simulink model "Test_SimFEAdapter"  (Simulink 7.4)
settings: Solver=FixedStepDiscrete  StartTime=0.0  StopTime=inf  FixedStep=samplePeriod  RelTol=1e-3  AbsTol=1e-6
PreLoadFcn:
  | initializeSimulation
InitFcn:
  | clear('all');
  | initializeSimulation;
values from neighbouring files (symbols this model uses):
  damperA = 0    [initializeSimulation.m]
  damperB = 0    [initializeSimulation.m]
  damperC = 0    [initializeSimulation.m]
  damperCanon = 1    [initializeSimulation.m]
  flowCanon = 3.85    [initializeSimulation.m]
  forceCanon = 1    [initializeSimulation.m]
  frictionA = 0    [initializeSimulation.m]
  frictionB = 0    [initializeSimulation.m]
  frictionC = 0    [initializeSimulation.m]
  gasConstant = 1.8    [initializeSimulation.m]
  lengthCanon = 1    [initializeSimulation.m]
  massA = 4.2    [initializeSimulation.m]
  massB = 2.5    [initializeSimulation.m]
  massC = 2.5    [initializeSimulation.m]
  massCanon = 0.002588    [initializeSimulation.m]
  maxDisplA = (stroke2A + endLength2A) * lengthCanon    (= 22)    [initializeSimulation.m]
  maxDisplB = (stroke2B + endLength2B) * lengthCanon    (= 42)    [initializeSimulation.m]
  maxDisplC = (stroke2C + endLength2C) * lengthCanon    (= 72)    [initializeSimulation.m]
  maxOilVolume = volume * (1 - (precharge/supplyPress)^(1/gasConstant))    (= 10.5071802963)    [initializeSimulation.m]
  maxVelocA = (maxFlowA * flowCanon / (area1A * areaCanon)) / velocCanon    [initializeSimulation.m]
  maxVelocB = (maxFlowB * flowCanon / (area1B * areaCanon)) / velocCanon    [initializeSimulation.m]
  maxVelocC = (maxFlowC * flowCanon / (area1C * areaCanon)) / velocCanon    [initializeSimulation.m]
  minDisplA = -(stroke1A + endLength1A) * lengthCanon    (= -22)    [initializeSimulation.m]
  minDisplB = -(stroke1B + endLength1B) * lengthCanon    (= -42)    [initializeSimulation.m]
  minDisplC = -(stroke1C + endLength1C) * lengthCanon    (= -72)    [initializeSimulation.m]
  minVelocA = -(maxFlowA * flowCanon / (area2A * areaCanon)) / velocCanon    [initializeSimulation.m]
  minVelocB = -(maxFlowB * flowCanon / (area2B * areaCanon)) / velocCanon    [initializeSimulation.m]
  minVelocC = -(maxFlowC * flowCanon / (area2C * areaCanon)) / velocCanon    [initializeSimulation.m]
  nAct = 8    [initializeSimulation.m]
  nAdcU = 12    [initializeSimulation.m]
  nDinp = 4    [initializeSimulation.m]
  nDout = 4    [initializeSimulation.m]
  nDucU = 8    [initializeSimulation.m]
  nEncU = 2    [initializeSimulation.m]
  precharge = 1000    [initializeSimulation.m]
  pumpFlow = 1e10    (= 10000000000)    [initializeSimulation.m]
  returnPress = 50    [initializeSimulation.m]
  staticForceA = 0    [initializeSimulation.m]
  staticForceB = 0    [initializeSimulation.m]
  staticForceC = 0    [initializeSimulation.m]
  supplyPress = 3000    [initializeSimulation.m]
  velocCanon = 1    [initializeSimulation.m]
  volume = accumVolume * accumNumber    (= 23)    [initializeSimulation.m]
  volumeCanon = 231    [initializeSimulation.m]
  yieldDisplA = 0.1    [initializeSimulation.m]
  yieldDisplB = 0.1    [initializeSimulation.m]
  yieldDisplC = 0.1    [initializeSimulation.m]
undefined symbols (not defined in the file or in its folder): DiscIntNeverNeededParam
(part 1 of 3)
settings Model: Creator=Andreas Schellenberg  LastModifiedBy=Andreas  ExtModeTrigMode=oneshot  ExtModeArmWhenConnect=off  ExtModeAutoUpdateStatusClock=off
settings DataIOCC: SaveOutput=off  SaveTime=off  SignalLoggingName=sigsOut
settings OptimizationCC: EnforceIntegerDowncast=off  InitFltsAndDblsToZero=on
settings DebuggingCC: SaveWithParameterizedLinksMsg=none  CheckSSInitialOutputMsg=off  SolverPrmCheckMsg=none  MultiTaskDSMMsg=warning  MultiTaskCondExecSysMsg=none  StrictBusMsg=None
settings HardwareCC: TargetUnknown=on
settings SFSimCC: SimCustomHeaderCode="#include \"PredictorCorrector.h\""  SimUserSources=PredictorCorrector.c
settings RTWCC: IncludeERTFirstTime=on
settings GRTTargetCC: TargetFcnLib=ansi_tfl_tmw.mat

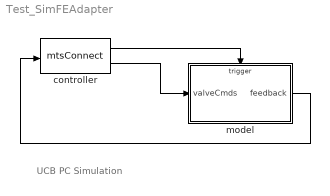
== system Test_SimFEAdapter ==
  note: UCB PC Simulation
  controller : S-Function  FunctionName=mtsConnect  Parameters='127.0.0.1',5002,nUDPInp,nUDPOut  EnableBusSupport=off
  model : Subsystem  TreatAsAtomicUnit=on
  wires:
  model/1(feedback) -> controller/1
  controller/2 -> model/1(valveCmds)
  controller/1 -> model/Trigger

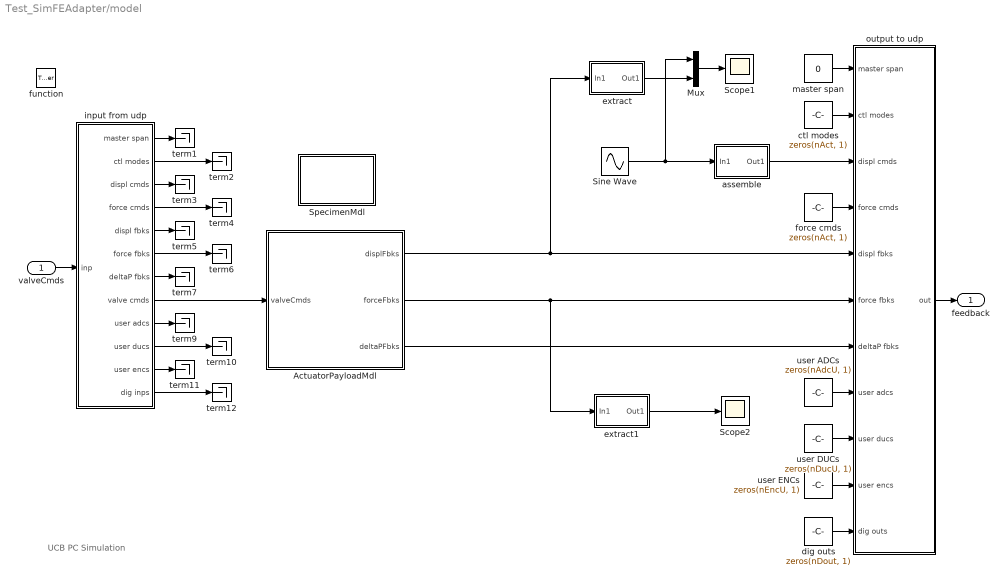
== system Test_SimFEAdapter/model ==
  note: UCB PC Simulation
  valveCmds : Inport  OutDataType=sfix(16)  OutScaling=2^0
  function : TriggerPort  TriggerType=function-call
  ActuatorPayloadMdl : Subsystem
  Mux : Mux  Inputs=2
  Scope1 : Scope
      settings: TimeRange=15  YMin=-1.5  YMax=1.5
  Scope2 : Scope
      settings: TimeRange=15  YMin=-6  YMax=8
  Sine Wave : Sin  Amplitude=1  Bias=0  Frequency=pi  Phase=0  Samples=10  Offset=0
  SpecimenMdl : Subsystem
      mask Display: fprintf('Test\nSpecimen');
  assemble : Subsystem  mask(to Actuators){id=1, size=nAct}
      mask prompts: id "Index Vector: id"; size "Vector Size: size"
      mask help: To select to which actuator(s) the signals are going to
      mask Display: disp('Assemble')
  ctl modes : Constant  Value=zeros(nAct, 1)  OutDataType=sfix(16)  OutScaling=2^0
  dig outs : Constant  Value=zeros(nDout, 1)  OutDataTypeMode=uint32  OutDataType=sfix(16)  OutScaling=2^0  OutDataTypeStr=uint32
  extract : Subsystem  mask(from Actuators){id=1, size=nAct}
      mask prompts: id "Index Vector: id"; size "Vector Size: size"
      mask help: To select from which actuator(s) the signals are coming from
      mask Display: disp('Extract')
  extract1 : Subsystem  mask(from Actuators){id=1, size=nAct}
      mask prompts: id "Index Vector: id"; size "Vector Size: size"
      mask help: To select from which actuator(s) the signals are coming from
      mask Display: disp('Extract')
  force cmds : Constant  Value=zeros(nAct, 1)  OutDataType=sfix(16)  OutScaling=2^0
  input from udp : Subsystem
  master span : Constant  Value=0  OutDataType=sfix(16)  OutScaling=2^0
  output to udp : Subsystem
  term{1..7,9..12} (11 alike) : Terminator
  user ADCs : Constant  Value=zeros(nAdcU, 1)  OutDataType=sfix(16)  OutScaling=2^0
  user DUCs : Constant  Value=zeros(nDucU, 1)  OutDataType=sfix(16)  OutScaling=2^0
  user ENCs : Constant  Value=zeros(nEncU, 1)  OutDataType=sfix(16)  OutScaling=2^0
  feedback : Outport  OutDataType=sfix(16)  OutScaling=2^0
  wires:
  input from udp/3(displ cmds) -> term3/1
  input from udp/1(master span) -> term1/1
  input from udp/6(force fbks) -> term6/1
  input from udp/10(user ducs) -> term10/1
  input from udp/12(dig inps) -> term12/1
  input from udp/2(ctl modes) -> term2/1
  input from udp/4(force cmds) -> term4/1
  input from udp/5(displ fbks) -> term5/1
  input from udp/7(deltaP fbks) -> term7/1
  input from udp/9(user adcs) -> term9/1
  input from udp/11(user encs) -> term11/1
  valveCmds/1 -> input from udp/1(inp)
  master span/1 -> output to udp/1(master span)
  ctl modes/1 -> output to udp/2(ctl modes)
  assemble/1(Out1) -> output to udp/3(displ cmds)
  force cmds/1 -> output to udp/4(force cmds)
  user ADCs/1 -> output to udp/8(user adcs)
  user DUCs/1 -> output to udp/9(user ducs)
  user ENCs/1 -> output to udp/10(user encs)
  dig outs/1 -> output to udp/11(dig outs)
  output to udp/1(out) -> feedback/1
  ActuatorPayloadMdl/1(displFbks) -> output to udp/5(displ fbks), extract/1(In1)
  ActuatorPayloadMdl/2(forceFbks) -> output to udp/6(force fbks), extract1/1(In1)
  ActuatorPayloadMdl/3(deltaPFbks) -> output to udp/7(deltaP fbks)
  input from udp/8(valve cmds) -> ActuatorPayloadMdl/1(valveCmds)
  Sine Wave/1 -> assemble/1(In1), Mux/1
  Mux/1 -> Scope1/1
  extract/1(Out1) -> Mux/2
  extract1/1(Out1) -> Scope2/1

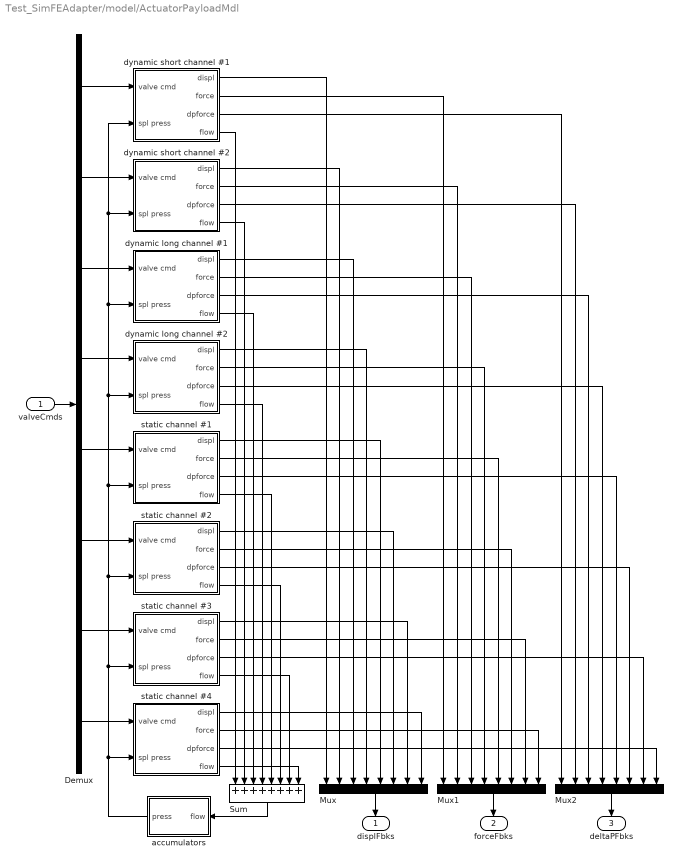
== system Test_SimFEAdapter/model/ActuatorPayloadMdl ==
  valveCmds : Inport  OutDataType=sfix(16)  OutScaling=2^0
  Demux : Demux  Outputs=nAct
  Mux : Mux  Inputs=nAct
  Mux1 : Mux  Inputs=nAct
  Mux2 : Mux  Inputs=nAct
  Sum : Sum  Inputs=++++++++  OutDataType=sfix(16)  OutScaling=2^0  SaturateOnIntegerOverflow=on
  accumulators : Subsystem
  dynamic long channel #1 : Subsystem
  dynamic long channel #2 : Subsystem
  dynamic short channel #1 : Subsystem
  dynamic short channel #2 : Subsystem
  static channel #1 : Subsystem
  static channel #2 : Subsystem
  static channel #3 : Subsystem
  static channel #4 : Subsystem
  displFbks : Outport  OutDataType=sfix(16)  OutScaling=2^0
  forceFbks : Outport  Port=2  OutDataType=sfix(16)  OutScaling=2^0
  deltaPFbks : Outport  Port=3  OutDataType=sfix(16)  OutScaling=2^0
  wires:
  Demux/1 -> dynamic short channel #1/1(valve cmd)
  Demux/3 -> dynamic long channel #1/1(valve cmd)
  Demux/2 -> dynamic short channel #2/1(valve cmd)
  dynamic short channel #1/4(flow) -> Sum/1
  dynamic short channel #2/4(flow) -> Sum/2
  dynamic long channel #1/4(flow) -> Sum/3
  Sum/1 -> accumulators/1(flow)
  Demux/4 -> dynamic long channel #2/1(valve cmd)
  Demux/5 -> static channel #1/1(valve cmd)
  Demux/6 -> static channel #2/1(valve cmd)
  Demux/7 -> static channel #3/1(valve cmd)
  Demux/8 -> static channel #4/1(valve cmd)
  dynamic long channel #2/4(flow) -> Sum/4
  static channel #1/4(flow) -> Sum/5
  static channel #2/4(flow) -> Sum/6
  static channel #3/4(flow) -> Sum/7
  static channel #4/4(flow) -> Sum/8
  accumulators/1(press) -> static channel #4/2(spl press), static channel #3/2(spl press), static channel #2/2(spl press), static channel #1/2(spl press), dynamic long channel #2/2(spl press), dynamic long channel #1/2(spl press), dynamic short channel #2/2(spl press), dynamic short channel #1/2(spl press)
  dynamic short channel #1/1(displ) -> Mux/1
  dynamic short channel #2/1(displ) -> Mux/2
  dynamic long channel #1/1(displ) -> Mux/3
  dynamic long channel #2/1(displ) -> Mux/4
  static channel #1/1(displ) -> Mux/5
  static channel #2/1(displ) -> Mux/6
  static channel #3/1(displ) -> Mux/7
  static channel #4/1(displ) -> Mux/8
  dynamic short channel #1/2(force) -> Mux1/1
  dynamic short channel #2/2(force) -> Mux1/2
  dynamic long channel #1/2(force) -> Mux1/3
  dynamic long channel #2/2(force) -> Mux1/4
  static channel #1/2(force) -> Mux1/5
  static channel #2/2(force) -> Mux1/6
  static channel #3/2(force) -> Mux1/7
  static channel #4/2(force) -> Mux1/8
  dynamic short channel #1/3(dpforce) -> Mux2/1
  dynamic short channel #2/3(dpforce) -> Mux2/2
  dynamic long channel #1/3(dpforce) -> Mux2/3
  dynamic long channel #2/3(dpforce) -> Mux2/4
  static channel #1/3(dpforce) -> Mux2/5
  static channel #2/3(dpforce) -> Mux2/6
  static channel #3/3(dpforce) -> Mux2/7
  static channel #4/3(dpforce) -> Mux2/8
  valveCmds/1 -> Demux/1
  Mux/1 -> displFbks/1
  Mux1/1 -> forceFbks/1
  Mux2/1 -> deltaPFbks/1

== system Test_SimFEAdapter/model/SpecimenMdl ==
  Scope3 : Scope
      settings: TimeRange=14  YMin=-2  YMax=2  SaveName=ScopeData2
  Specimen #1 : S-Function  FunctionName=SFun_SimFEAdapter  Parameters=ipAddr,ipPort,dataSize  EnableBusSupport=off  mask(GenericClient Element){ipAddr=127.0.0.1, ipPort=44000, dataSize=256}
      mask prompts: ipAddr "IP Address of Adapter Element"; ipPort "IP Port Number of Adapter Element"; dataSize "Size of Data Arrays"
      mask Display: disp('SimFE\nAdapter');
  Terminator : Terminator
  assemble1 : Subsystem  mask(to Actuators){id=1, size=nAct}
      mask prompts: id "Index Vector: id"; size "Vector Size: size"
      mask help: To select to which actuator(s) the signals are going to
      mask Display: disp('Assemble')
  assemble2 : Subsystem  mask(to Actuators){id=1, size=nAct}
      mask prompts: id "Index Vector: id"; size "Vector Size: size"
      mask help: To select to which actuator(s) the signals are going to
      mask Display: disp('Assemble')
  extract2 : Subsystem  mask(from Actuators){id=1, size=nAct}
      mask prompts: id "Index Vector: id"; size "Vector Size: size"
      mask help: To select from which actuator(s) the signals are coming from
      mask Display: disp('Extract')
  from Actuators : Subsystem
  to LoadCells : Subsystem
  wires:
  from Actuators/1(ctrlDisp) -> extract2/1(In1)
  extract2/1(Out1) -> Specimen #1/1
  Specimen #1/1 -> assemble2/1(In1)
  Specimen #1/2 -> assemble1/1(In1), Scope3/1
  assemble2/1(Out1) -> Terminator/1
  assemble1/1(Out1) -> to LoadCells/1(daqForce)

== system Test_SimFEAdapter/model/assemble ==
  In1 : Inport  OutDataType=sfix(16)  OutScaling=2^0
  Assignment : Assignment  OutputInitialize=Specify size for each dimension in table  IndexOptions=Index vector (port)  Indices=1  OutputSizes=nAct
  Constant : Constant  Value=id  OutDataType=sfix(16)  OutScaling=2^0
  Out1 : Outport  OutDataType=sfix(16)  OutScaling=2^0
  wires:
  Constant/1 -> Assignment/2
  Assignment/1 -> Out1/1
  In1/1 -> Assignment/1

== system Test_SimFEAdapter/model/extract ==
  In1 : Inport  OutDataType=sfix(16)  OutScaling=2^0
  Selector : Selector  InputPortWidth=size  IndexOptions=Index vector (dialog)  Indices=id  OutputSizes=1
  Out1 : Outport  OutDataType=sfix(16)  OutScaling=2^0
  wires:
  Selector/1 -> Out1/1
  In1/1 -> Selector/1

== system Test_SimFEAdapter/model/extract1 ==
  In1 : Inport  OutDataType=sfix(16)  OutScaling=2^0
  Selector : Selector  InputPortWidth=size  IndexOptions=Index vector (dialog)  Indices=id  OutputSizes=1
  Out1 : Outport  OutDataType=sfix(16)  OutScaling=2^0
  wires:
  Selector/1 -> Out1/1
  In1/1 -> Selector/1

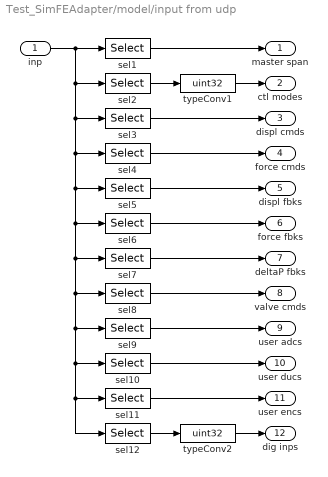
== system Test_SimFEAdapter/model/input from udp ==
  inp : Inport  OutDataType=sfix(16)  OutScaling=2^0
  sel1 : Selector  InputPortWidth=nUDPOut  IndexOptions=Index vector (dialog)  Indices=[0]+1  OutputSizes=1
  sel10 : Selector  InputPortWidth=nUDPOut  IndexOptions=Index vector (dialog)  Indices=[1:nDucU]+1+7*nAct+nAdcU  OutputSizes=1
  sel11 : Selector  InputPortWidth=nUDPOut  IndexOptions=Index vector (dialog)  Indices=[1:nEncU]+1+7*nAct+nAdcU+nDucU  OutputSizes=1
  sel12 : Selector  InputPortWidth=nUDPOut  IndexOptions=Index vector (dialog)  Indices=[1:nDinp]+1+7*nAct+nAdcU+nDucU+nEncU  OutputSizes=1
  sel2 : Selector  InputPortWidth=nUDPOut  IndexOptions=Index vector (dialog)  Indices=[1:nAct]+1+0*nAct  OutputSizes=1
  sel3 : Selector  InputPortWidth=nUDPOut  IndexOptions=Index vector (dialog)  Indices=[1:nAct]+1+1*nAct  OutputSizes=1
  sel4 : Selector  InputPortWidth=nUDPOut  IndexOptions=Index vector (dialog)  Indices=[1:nAct]+1+2*nAct  OutputSizes=1
  sel5 : Selector  InputPortWidth=nUDPOut  IndexOptions=Index vector (dialog)  Indices=[1:nAct]+1+3*nAct  OutputSizes=1
  sel6 : Selector  InputPortWidth=nUDPOut  IndexOptions=Index vector (dialog)  Indices=[1:nAct]+1+4*nAct  OutputSizes=1
  sel7 : Selector  InputPortWidth=nUDPOut  IndexOptions=Index vector (dialog)  Indices=[1:nAct]+1+5*nAct  OutputSizes=1
  sel8 : Selector  InputPortWidth=nUDPOut  IndexOptions=Index vector (dialog)  Indices=[1:nAct]+1+6*nAct  OutputSizes=1
  sel9 : Selector  InputPortWidth=nUDPOut  IndexOptions=Index vector (dialog)  Indices=[1:nAdcU]+1+7*nAct  OutputSizes=1
  typeConv1 : DataTypeConversion  OutDataTypeMode=uint32  OutDataType=sfix(16)  OutScaling=2^0  OutDataTypeStr=uint32  SaturateOnIntegerOverflow=on  RndMeth=Zero
  typeConv2 : DataTypeConversion  OutDataTypeMode=uint32  OutDataType=sfix(16)  OutScaling=2^0  OutDataTypeStr=uint32  SaturateOnIntegerOverflow=on  RndMeth=Zero
  master span : Outport  OutDataType=sfix(16)  OutScaling=2^0
  ctl modes : Outport  Port=2  OutDataType=sfix(16)  OutScaling=2^0
  displ cmds : Outport  Port=3  OutDataType=sfix(16)  OutScaling=2^0
  force cmds : Outport  Port=4  OutDataType=sfix(16)  OutScaling=2^0
  displ fbks : Outport  Port=5  OutDataType=sfix(16)  OutScaling=2^0
  force fbks : Outport  Port=6  OutDataType=sfix(16)  OutScaling=2^0
  deltaP fbks : Outport  Port=7  OutDataType=sfix(16)  OutScaling=2^0
  valve cmds : Outport  Port=8  OutDataType=sfix(16)  OutScaling=2^0
  user adcs : Outport  Port=9  OutDataType=sfix(16)  OutScaling=2^0
  user ducs : Outport  Port=10  OutDataType=sfix(16)  OutScaling=2^0
  user encs : Outport  Port=11  OutDataType=sfix(16)  OutScaling=2^0
  dig inps : Outport  Port=12  OutDataType=sfix(16)  OutScaling=2^0
  wires:
  sel1/1 -> master span/1
  sel2/1 -> typeConv1/1
  sel3/1 -> displ cmds/1
  sel4/1 -> force cmds/1
  sel5/1 -> displ fbks/1
  sel6/1 -> force fbks/1
  sel7/1 -> deltaP fbks/1
  sel8/1 -> valve cmds/1
  sel9/1 -> user adcs/1
  sel10/1 -> user ducs/1
  sel11/1 -> user encs/1
  sel12/1 -> typeConv2/1
  inp/1 -> sel1/1, sel2/1, sel3/1, sel11/1, sel12/1, sel10/1, sel9/1, sel8/1, sel7/1, sel6/1, sel5/1, sel4/1
  typeConv1/1 -> ctl modes/1
  typeConv2/1 -> dig inps/1

== system Test_SimFEAdapter/model/output to udp ==
  master span : Inport  OutDataType=sfix(16)  OutScaling=2^0
  ctl modes : Inport  Port=2  OutDataType=sfix(16)  OutScaling=2^0
  displ cmds : Inport  Port=3  OutDataType=sfix(16)  OutScaling=2^0
  force cmds : Inport  Port=4  OutDataType=sfix(16)  OutScaling=2^0
  displ fbks : Inport  Port=5  OutDataType=sfix(16)  OutScaling=2^0
  force fbks : Inport  Port=6  OutDataType=sfix(16)  OutScaling=2^0
  deltaP fbks : Inport  Port=7  OutDataType=sfix(16)  OutScaling=2^0
  user adcs : Inport  Port=8  OutDataType=sfix(16)  OutScaling=2^0
  user ducs : Inport  Port=9  OutDataType=sfix(16)  OutScaling=2^0
  user encs : Inport  Port=10  OutDataType=sfix(16)  OutScaling=2^0
  dig outs : Inport  Port=11  OutDataType=sfix(16)  OutScaling=2^0
  Mux : Mux  Inputs=11
  typeConv1 : DataTypeConversion  OutDataTypeMode=double  OutDataType=sfix(16)  OutScaling=2^0  OutDataTypeStr=double  SaturateOnIntegerOverflow=on  RndMeth=Zero
  typeConv2 : DataTypeConversion  OutDataTypeMode=double  OutDataType=sfix(16)  OutScaling=2^0  OutDataTypeStr=double  SaturateOnIntegerOverflow=on  RndMeth=Zero
  out : Outport  OutDataType=sfix(16)  OutScaling=2^0
  wires:
  typeConv2/1 -> Mux/11
  dig outs/1 -> typeConv2/1
  user encs/1 -> Mux/10
  user ducs/1 -> Mux/9
  user adcs/1 -> Mux/8
  deltaP fbks/1 -> Mux/7
  force fbks/1 -> Mux/6
  displ fbks/1 -> Mux/5
  force cmds/1 -> Mux/4
  master span/1 -> Mux/1
  displ cmds/1 -> Mux/3
  ctl modes/1 -> typeConv1/1
  Mux/1 -> out/1
  typeConv1/1 -> Mux/2

== system Test_SimFEAdapter/model/ActuatorPayloadMdl/accumulators ==
  flow : Inport  OutDataType=sfix(16)  OutScaling=2^0
  Sum : Sum  Inputs=+-|  OutDataType=sfix(16)  OutScaling=2^0  SaturateOnIntegerOverflow=on  InputSameDT=on  OutDataTypeStr=Inherit: Same as first input
  Sum1 : Sum  Inputs=+-|  OutDataType=sfix(16)  OutScaling=2^0  SaturateOnIntegerOverflow=on  InputSameDT=on  OutDataTypeStr=Inherit: Same as first input
  bottle volume : Constant  Value=volume*volumeCanon  OutDataType=sfix(16)  OutScaling=2^0
  flowCanon : Gain  Gain=flowCanon  ParameterDataType=sfix(16)  ParameterScaling=2^0  OutDataType=sfix(16)  OutScaling=2^0  SaturateOnIntegerOverflow=on  OutDataTypeStr=Inherit: Same as input  ParamDataTypeStr=Inherit: Same as input
  gas constant : Constant  Value=gasConstant  OutDataType=sfix(16)  OutScaling=2^0
  initial condition : UnitDelay  X0=supplyPress  SampleTime=-1
  integrator : DiscreteIntegrator  InitialCondition=maxOilVolume*volumeCanon  SampleTime=-1  OutDataType=sfix(16)  OutScaling=2^0  LimitOutput=on  UpperSaturationLimit=maxOilVolume*volumeCanon  LowerSaturationLimit=0  ICPrevOutput=DiscIntNeverNeededParam  ICPrevScaledInput=DiscIntNeverNeededParam
  power : Math  Operator=pow  OutDataType=sfix(16)  OutScaling=2^0  SaturateOnIntegerOverflow=on
  precharge : Gain  Gain=precharge  ParameterDataType=sfix(16)  ParameterScaling=2^0  OutDataType=sfix(16)  OutScaling=2^0  SaturateOnIntegerOverflow=on  OutDataTypeStr=Inherit: Same as input  ParamDataTypeStr=Inherit: Same as input
  pump flow : Constant  Value=pumpFlow  OutDataType=sfix(16)  OutScaling=2^0
  quotient : Product  Inputs=*/  OutDataType=sfix(16)  OutScaling=2^0  SaturateOnIntegerOverflow=on  InputSameDT=on  OutDataTypeStr=Inherit: Same as first input
  press : Outport  OutDataType=sfix(16)  OutScaling=2^0
  wires:
  initial condition/1 -> press/1
  flowCanon/1 -> integrator/1
  flow/1 -> Sum/2
  integrator/1 -> Sum1/2  "current oil volume"
  quotient/1 -> power/1
  Sum1/1 -> quotient/2  "current gas volume"
  precharge/1 -> initial condition/1
  power/1 -> precharge/1
  gas constant/1 -> power/2
  bottle volume/1 -> quotient/1, Sum1/1
  Sum/1 -> flowCanon/1
  pump flow/1 -> Sum/1

== system Test_SimFEAdapter/model/ActuatorPayloadMdl/dynamic long channel #1 ==
  valve cmd : Inport  OutDataType=sfix(16)  OutScaling=2^0
  spl press : Inport  Port=2  OutDataType=sfix(16)  OutScaling=2^0
  actuator/valve  model : Subsystem
      mask Type: Inverse Actuator
  payload : Subsystem
  return pressure : Constant  Value=returnPress  OutDataType=sfix(16)  OutScaling=2^0
  displ : Outport  OutDataType=sfix(16)  OutScaling=2^0
  force : Outport  Port=2  OutDataType=sfix(16)  OutScaling=2^0
  dpforce : Outport  Port=3  OutDataType=sfix(16)  OutScaling=2^0
  flow : Outport  Port=4  OutDataType=sfix(16)  OutScaling=2^0
  wires:
  payload/2(veloc) -> actuator/valve  model/3(veloc)
  payload/1(displ) -> displ/1, actuator/valve  model/2(displ)
  valve cmd/1 -> actuator/valve  model/1(cmd)
  return pressure/1 -> actuator/valve  model/5(rtn press)
  spl press/1 -> actuator/valve  model/4(spl press)
  actuator/valve  model/2(flow) -> flow/1
  actuator/valve  model/1(force) -> force/1, dpforce/1, payload/1(force)

== system Test_SimFEAdapter/model/ActuatorPayloadMdl/dynamic long channel #2 ==
  valve cmd : Inport  OutDataType=sfix(16)  OutScaling=2^0
  spl press : Inport  Port=2  OutDataType=sfix(16)  OutScaling=2^0
  actuator/valve  model : Subsystem
      mask Type: Inverse Actuator
  payload : Subsystem
  return pressure : Constant  Value=returnPress  OutDataType=sfix(16)  OutScaling=2^0
  displ : Outport  OutDataType=sfix(16)  OutScaling=2^0
  force : Outport  Port=2  OutDataType=sfix(16)  OutScaling=2^0
  dpforce : Outport  Port=3  OutDataType=sfix(16)  OutScaling=2^0
  flow : Outport  Port=4  OutDataType=sfix(16)  OutScaling=2^0
  wires:
  actuator/valve  model/1(force) -> dpforce/1, force/1, payload/1(force)
  actuator/valve  model/2(flow) -> flow/1
  spl press/1 -> actuator/valve  model/4(spl press)
  return pressure/1 -> actuator/valve  model/5(rtn press)
  valve cmd/1 -> actuator/valve  model/1(cmd)
  payload/1(displ) -> actuator/valve  model/2(displ), displ/1
  payload/2(veloc) -> actuator/valve  model/3(veloc)

== system Test_SimFEAdapter/model/ActuatorPayloadMdl/dynamic short channel #1 ==
  valve cmd : Inport  OutDataType=sfix(16)  OutScaling=2^0
  spl press : Inport  Port=2  OutDataType=sfix(16)  OutScaling=2^0
  actuator/valve  model : Subsystem
      mask Type: Inverse Actuator
  payload : Subsystem
  return pressure : Constant  Value=returnPress  OutDataType=sfix(16)  OutScaling=2^0
  displ : Outport  OutDataType=sfix(16)  OutScaling=2^0
  force : Outport  Port=2  OutDataType=sfix(16)  OutScaling=2^0
  dpforce : Outport  Port=3  OutDataType=sfix(16)  OutScaling=2^0
  flow : Outport  Port=4  OutDataType=sfix(16)  OutScaling=2^0
  wires:
  actuator/valve  model/1(force) -> dpforce/1, force/1, payload/1(force)
  actuator/valve  model/2(flow) -> flow/1
  spl press/1 -> actuator/valve  model/4(spl press)
  return pressure/1 -> actuator/valve  model/5(rtn press)
  valve cmd/1 -> actuator/valve  model/1(cmd)
  payload/1(displ) -> actuator/valve  model/2(displ), displ/1
  payload/2(veloc) -> actuator/valve  model/3(veloc)

== system Test_SimFEAdapter/model/ActuatorPayloadMdl/dynamic short channel #2 ==
  valve cmd : Inport  OutDataType=sfix(16)  OutScaling=2^0
  spl press : Inport  Port=2  OutDataType=sfix(16)  OutScaling=2^0
  actuator/valve  model : Subsystem
      mask Type: Inverse Actuator
  payload : Subsystem
  return pressure : Constant  Value=returnPress  OutDataType=sfix(16)  OutScaling=2^0
  displ : Outport  OutDataType=sfix(16)  OutScaling=2^0
  force : Outport  Port=2  OutDataType=sfix(16)  OutScaling=2^0
  dpforce : Outport  Port=3  OutDataType=sfix(16)  OutScaling=2^0
  flow : Outport  Port=4  OutDataType=sfix(16)  OutScaling=2^0
  wires:
  actuator/valve  model/1(force) -> dpforce/1, force/1, payload/1(force)
  actuator/valve  model/2(flow) -> flow/1
  spl press/1 -> actuator/valve  model/4(spl press)
  return pressure/1 -> actuator/valve  model/5(rtn press)
  valve cmd/1 -> actuator/valve  model/1(cmd)
  payload/1(displ) -> actuator/valve  model/2(displ), displ/1
  payload/2(veloc) -> actuator/valve  model/3(veloc)

== system Test_SimFEAdapter/model/ActuatorPayloadMdl/static channel #1 ==
  valve cmd : Inport  OutDataType=sfix(16)  OutScaling=2^0
  spl press : Inport  Port=2  OutDataType=sfix(16)  OutScaling=2^0
  actuator/valve  model : Subsystem
      mask Type: Inverse Actuator
  payload : Subsystem
  return pressure : Constant  Value=returnPress  OutDataType=sfix(16)  OutScaling=2^0
  displ : Outport  OutDataType=sfix(16)  OutScaling=2^0
  force : Outport  Port=2  OutDataType=sfix(16)  OutScaling=2^0
  dpforce : Outport  Port=3  OutDataType=sfix(16)  OutScaling=2^0
  flow : Outport  Port=4  OutDataType=sfix(16)  OutScaling=2^0
  wires:
  payload/2(veloc) -> actuator/valve  model/3(veloc)
  payload/1(displ) -> displ/1, actuator/valve  model/2(displ)
  valve cmd/1 -> actuator/valve  model/1(cmd)
  return pressure/1 -> actuator/valve  model/5(rtn press)
  spl press/1 -> actuator/valve  model/4(spl press)
  actuator/valve  model/2(flow) -> flow/1
  actuator/valve  model/1(force) -> force/1, dpforce/1, payload/1(force)

== system Test_SimFEAdapter/model/ActuatorPayloadMdl/static channel #2 ==
  valve cmd : Inport  OutDataType=sfix(16)  OutScaling=2^0
  spl press : Inport  Port=2  OutDataType=sfix(16)  OutScaling=2^0
  actuator/valve  model : Subsystem
      mask Type: Inverse Actuator
  payload : Subsystem
  return pressure : Constant  Value=returnPress  OutDataType=sfix(16)  OutScaling=2^0
  displ : Outport  OutDataType=sfix(16)  OutScaling=2^0
  force : Outport  Port=2  OutDataType=sfix(16)  OutScaling=2^0
  dpforce : Outport  Port=3  OutDataType=sfix(16)  OutScaling=2^0
  flow : Outport  Port=4  OutDataType=sfix(16)  OutScaling=2^0
  wires:
  actuator/valve  model/1(force) -> dpforce/1, force/1, payload/1(force)
  actuator/valve  model/2(flow) -> flow/1
  spl press/1 -> actuator/valve  model/4(spl press)
  return pressure/1 -> actuator/valve  model/5(rtn press)
  valve cmd/1 -> actuator/valve  model/1(cmd)
  payload/1(displ) -> actuator/valve  model/2(displ), displ/1
  payload/2(veloc) -> actuator/valve  model/3(veloc)

== system Test_SimFEAdapter/model/ActuatorPayloadMdl/static channel #3 ==
  valve cmd : Inport  OutDataType=sfix(16)  OutScaling=2^0
  spl press : Inport  Port=2  OutDataType=sfix(16)  OutScaling=2^0
  actuator/valve  model : Subsystem
      mask Type: Inverse Actuator
  payload : Subsystem
  return pressure : Constant  Value=returnPress  OutDataType=sfix(16)  OutScaling=2^0
  displ : Outport  OutDataType=sfix(16)  OutScaling=2^0
  force : Outport  Port=2  OutDataType=sfix(16)  OutScaling=2^0
  dpforce : Outport  Port=3  OutDataType=sfix(16)  OutScaling=2^0
  flow : Outport  Port=4  OutDataType=sfix(16)  OutScaling=2^0
  wires:
  payload/2(veloc) -> actuator/valve  model/3(veloc)
  payload/1(displ) -> displ/1, actuator/valve  model/2(displ)
  valve cmd/1 -> actuator/valve  model/1(cmd)
  return pressure/1 -> actuator/valve  model/5(rtn press)
  spl press/1 -> actuator/valve  model/4(spl press)
  actuator/valve  model/2(flow) -> flow/1
  actuator/valve  model/1(force) -> force/1, dpforce/1, payload/1(force)

== system Test_SimFEAdapter/model/ActuatorPayloadMdl/static channel #4 ==
  valve cmd : Inport  OutDataType=sfix(16)  OutScaling=2^0
  spl press : Inport  Port=2  OutDataType=sfix(16)  OutScaling=2^0
  actuator/valve  model : Subsystem
      mask Type: Inverse Actuator
  payload : Subsystem
  return pressure : Constant  Value=returnPress  OutDataType=sfix(16)  OutScaling=2^0
  displ : Outport  OutDataType=sfix(16)  OutScaling=2^0
  force : Outport  Port=2  OutDataType=sfix(16)  OutScaling=2^0
  dpforce : Outport  Port=3  OutDataType=sfix(16)  OutScaling=2^0
  flow : Outport  Port=4  OutDataType=sfix(16)  OutScaling=2^0
  wires:
  actuator/valve  model/1(force) -> dpforce/1, force/1, payload/1(force)
  actuator/valve  model/2(flow) -> flow/1
  spl press/1 -> actuator/valve  model/4(spl press)
  return pressure/1 -> actuator/valve  model/5(rtn press)
  valve cmd/1 -> actuator/valve  model/1(cmd)
  payload/1(displ) -> actuator/valve  model/2(displ), displ/1
  payload/2(veloc) -> actuator/valve  model/3(veloc)

== system Test_SimFEAdapter/model/SpecimenMdl/assemble1 ==
  In1 : Inport  OutDataType=sfix(16)  OutScaling=2^0
  Assignment : Assignment  OutputInitialize=Specify size for each dimension in table  IndexOptions=Index vector (port)  Indices=1  OutputSizes=nAct
  Constant : Constant  Value=id  OutDataType=sfix(16)  OutScaling=2^0
  Out1 : Outport  OutDataType=sfix(16)  OutScaling=2^0
  wires:
  Constant/1 -> Assignment/2
  Assignment/1 -> Out1/1
  In1/1 -> Assignment/1

== system Test_SimFEAdapter/model/SpecimenMdl/assemble2 ==
  In1 : Inport  OutDataType=sfix(16)  OutScaling=2^0
  Assignment : Assignment  OutputInitialize=Specify size for each dimension in table  IndexOptions=Index vector (port)  Indices=1  OutputSizes=nAct
  Constant : Constant  Value=id  OutDataType=sfix(16)  OutScaling=2^0
  Out1 : Outport  OutDataType=sfix(16)  OutScaling=2^0
  wires:
  Constant/1 -> Assignment/2
  Assignment/1 -> Out1/1
  In1/1 -> Assignment/1

== system Test_SimFEAdapter/model/SpecimenMdl/extract2 ==
  In1 : Inport  OutDataType=sfix(16)  OutScaling=2^0
  Selector : Selector  InputPortWidth=size  IndexOptions=Index vector (dialog)  Indices=id  OutputSizes=1
  Out1 : Outport  OutDataType=sfix(16)  OutScaling=2^0
  wires:
  Selector/1 -> Out1/1
  In1/1 -> Selector/1

== system Test_SimFEAdapter/model/SpecimenMdl/from Actuators ==
  Bus Creator : BusCreator  Inputs=8
  ctrlDisp : Outport
  wires:
  [ch1a] -> Bus Creator/1
  [ch2a] -> Bus Creator/2
  [ch3a] -> Bus Creator/3
  [ch4a] -> Bus Creator/4
  [ch5a] -> Bus Creator/5
  [ch6a] -> Bus Creator/6
  [ch7a] -> Bus Creator/7
  [ch8a] -> Bus Creator/8
  Bus Creator/1 -> ctrlDisp/1

== system Test_SimFEAdapter/model/SpecimenMdl/to LoadCells ==
  daqForce : Inport
  Demux : Demux  Outputs=8
  tag scope: ch1b=global, ch2b=global, ch3b=global, ch4b=global, ch5b=global, ch6b=global, ch7b=global, ch8b=global
  wires:
  Demux/1 -> [ch1b]
  Demux/2 -> [ch2b]
  Demux/3 -> [ch3b]
  Demux/4 -> [ch4b]
  Demux/5 -> [ch5b]
  Demux/6 -> [ch6b]
  Demux/7 -> [ch7b]
  Demux/8 -> [ch8b]
  daqForce/1 -> Demux/1

== system Test_SimFEAdapter/model/ActuatorPayloadMdl/dynamic long channel #1/actuator/valve  model ==
  note: Note: "1" and "2" denote actuator
      | cylinders on either side of the
      | actuator piston.  With positive
      | valve drive, oil is ported into
      | cylinder 1, resulting in positive
      | displacement.
  note: Auxiliary diagnostic output vector:
      | 1:   valve opening
      | 2:   C1 pressure
      | 3:   C2 pressure
      | 4:   delta pressure
      | 5:   force
      | 6:   velocity
      | 7:   C1 flow
      | 8:   C2 flow
      | 9:   total flow
      | 10: kinematic flow
      | 11: compressibility flow
      | 12: leakage flow
  note: Parameter vector:
      | 1:   oil bulk modulus (force/displ^2)
      | 2:   servovalve delay (sec)
      | 3:   servovalve overlap
      | 4:   rated pressure (force/displ^2)
      | 5:   rated flow at rated pressure (displ^3/sec)
      | 6:   nominal flow at rated pressure (displ^3/sec)
      | 7:   actuator piston area 1 (displ^2)
      | 8:   actuator piston area 2 (displ^2)
      | 9:   actuator usable stroke 1 (displ)
      | 10: actuator usable stroke 2 (displ)
      | 11: actuator end cushion length 1 (displ)
      | 12: actuator end cushion length 2 (displ)
      | 13: actuator parasitic damping factor
      | 14: cross-chamber leakage factor (flow/press)
      | 15: ratio port openings according to area
      | 16: sample period (sec)
      |
      | Conversion factors used for converting
      | signals from external (user) to internal
      | (canonical) units:
      |
      | 17: displacement
      | 18: velocity
      | 19: force
      | 20: pressure
      | 21: flow
  cmd : Inport  OutDataType=sfix(16)  OutScaling=2^0
  displ : Inport  Port=2  OutDataType=sfix(16)  OutScaling=2^0
  veloc : Inport  Port=3  OutDataType=sfix(16)  OutScaling=2^0
  spl press : Inport  Port=4  OutDataType=sfix(16)  OutScaling=2^0
  rtn press : Inport  Port=5  OutDataType=sfix(16)  OutScaling=2^0
  abs : Abs  SaturateOnIntegerOverflow=on
  actuator : S-Function  FunctionName=actuator  Parameters=actParamsB  EnableBusSupport=off
  total flow sel : Selector  InputPortWidth=12  IndexOptions=Index vector (dialog)  Indices=9  OutputSizes=1
  force : Outport  OutDataType=sfix(16)  OutScaling=2^0
  flow : Outport  Port=2  OutDataType=sfix(16)  OutScaling=2^0
  wires:
  veloc/1 -> actuator/3
  displ/1 -> actuator/2
  actuator/1 -> force/1
  cmd/1 -> actuator/1
  rtn press/1 -> actuator/5
  spl press/1 -> actuator/4
  total flow sel/1 -> abs/1
  actuator/2 -> total flow sel/1
  abs/1 -> flow/1

== system Test_SimFEAdapter/model/ActuatorPayloadMdl/dynamic long channel #1/payload ==
  force : Inport  OutDataType=sfix(16)  OutScaling=2^0
  Sum : Sum  Inputs=+----  OutDataType=sfix(16)  OutScaling=2^0  SaturateOnIntegerOverflow=on  InputSameDT=on  OutDataTypeStr=Inherit: Same as first input
  damper : Gain  Gain=damperB*damperCanon  ParameterDataType=sfix(16)  ParameterScaling=2^0  OutDataType=sfix(16)  OutScaling=2^0  SaturateOnIntegerOverflow=on  OutDataTypeStr=Inherit: Same as input  ParamDataTypeStr=Inherit: Same as input
  div : Product  Inputs=*/  OutDataType=sfix(16)  OutScaling=2^0  SaturateOnIntegerOverflow=on  InputSameDT=on  OutDataTypeStr=Inherit: Same as first input
  double integrator : Subsystem
  friction : Subsystem  mask{friction=frictionB*forceCanon, yieldDispl=yieldDisplB*lengthCanon, hysteresis=0}
      mask prompts: friction "Sliding friction"; yieldDispl "Equiv. yield displacement (in)"; hysteresis "Hysteresis constant"
  mass : Constant  Value=massB*massCanon  OutDataType=sfix(16)  OutScaling=2^0
  static force : Constant  Value=staticForceB*forceCanon  OutDataType=sfix(16)  OutScaling=2^0
  term1 : Terminator
  unit dly : UnitDelay  SampleTime=-1
  unit dly1 : UnitDelay  SampleTime=-1
  veloc units : Gain  Gain=1/velocCanon  ParameterDataType=sfix(16)  ParameterScaling=2^0  OutDataType=sfix(16)  OutScaling=2^0  SaturateOnIntegerOverflow=on  OutDataTypeStr=Inherit: Same as input  ParamDataTypeStr=Inherit: Same as input
  displ : Outport  OutDataType=sfix(16)  OutScaling=2^0
  veloc : Outport  Port=2  OutDataType=sfix(16)  OutScaling=2^0
  tag scope: ch3a=global
  wires:
  friction/1(force) -> Sum/2  "friction force"
  veloc units/1 -> veloc/1
  Sum/1 -> div/1  "inertial force"
  force/1 -> Sum/1  "total force"
  mass/1 -> div/2
  double integrator/3(acc) -> term1/1
  div/1 -> double integrator/1(accel)
  double integrator/1(displ) -> displ/1, unit dly/1
  double integrator/2(veloc) -> veloc units/1, friction/1(veloc), unit dly1/1
  static force/1 -> Sum/5  "static force"
  damper/1 -> Sum/4  "damper force"
  unit dly1/1 -> damper/1
  [ch3b] -> Sum/3  "spring force"
  unit dly/1 -> [ch3a]

== system Test_SimFEAdapter/model/ActuatorPayloadMdl/dynamic long channel #2/actuator/valve  model ==
  note: Auxiliary diagnostic output vector:
      | 1:   valve opening
      | 2:   C1 pressure
      | 3:   C2 pressure
      | 4:   delta pressure
      | 5:   force
      | 6:   velocity
      | 7:   C1 flow
      | 8:   C2 flow
      | 9:   total flow
      | 10: kinematic flow
      | 11: compressibility flow
      | 12: leakage flow
  note: Note: "1" and "2" denote actuator
      | cylinders on either side of the
      | actuator piston.  With positive
      | valve drive, oil is ported into
      | cylinder 1, resulting in positive
      | displacement.
  note: Parameter vector:
      | 1:   oil bulk modulus (force/displ^2)
      | 2:   servovalve delay (sec)
      | 3:   servovalve overlap
      | 4:   rated pressure (force/displ^2)
      | 5:   rated flow at rated pressure (displ^3/sec)
      | 6:   nominal flow at rated pressure (displ^3/sec)
      | 7:   actuator piston area 1 (displ^2)
      | 8:   actuator piston area 2 (displ^2)
      | 9:   actuator usable stroke 1 (displ)
      | 10: actuator usable stroke 2 (displ)
      | 11: actuator end cushion length 1 (displ)
      | 12: actuator end cushion length 2 (displ)
      | 13: actuator parasitic damping factor
      | 14: cross-chamber leakage factor (flow/press)
      | 15: ratio port openings according to area
      | 16: sample period (sec)
      |
      | Conversion factors used for converting
      | signals from external (user) to internal
      | (canonical) units:
      |
      | 17: displacement
      | 18: velocity
      | 19: force
      | 20: pressure
      | 21: flow
  cmd : Inport  OutDataType=sfix(16)  OutScaling=2^0
  displ : Inport  Port=2  OutDataType=sfix(16)  OutScaling=2^0
  veloc : Inport  Port=3  OutDataType=sfix(16)  OutScaling=2^0
  spl press : Inport  Port=4  OutDataType=sfix(16)  OutScaling=2^0
  rtn press : Inport  Port=5  OutDataType=sfix(16)  OutScaling=2^0
  abs : Abs  SaturateOnIntegerOverflow=on
  actuator : S-Function  FunctionName=actuator  Parameters=actParamsB  EnableBusSupport=off
  total flow sel : Selector  InputPortWidth=12  IndexOptions=Index vector (dialog)  Indices=9  OutputSizes=1
  force : Outport  OutDataType=sfix(16)  OutScaling=2^0
  flow : Outport  Port=2  OutDataType=sfix(16)  OutScaling=2^0
  wires:
  abs/1 -> flow/1
  actuator/2 -> total flow sel/1
  total flow sel/1 -> abs/1
  spl press/1 -> actuator/4
  rtn press/1 -> actuator/5
  cmd/1 -> actuator/1
  actuator/1 -> force/1
  displ/1 -> actuator/2
  veloc/1 -> actuator/3

== system Test_SimFEAdapter/model/ActuatorPayloadMdl/dynamic long channel #2/payload ==
  force : Inport  OutDataType=sfix(16)  OutScaling=2^0
  Sum : Sum  Inputs=+----  OutDataType=sfix(16)  OutScaling=2^0  SaturateOnIntegerOverflow=on  InputSameDT=on  OutDataTypeStr=Inherit: Same as first input
  damper : Gain  Gain=damperB*damperCanon  ParameterDataType=sfix(16)  ParameterScaling=2^0  OutDataType=sfix(16)  OutScaling=2^0  SaturateOnIntegerOverflow=on  OutDataTypeStr=Inherit: Same as input  ParamDataTypeStr=Inherit: Same as input
  div : Product  Inputs=*/  OutDataType=sfix(16)  OutScaling=2^0  SaturateOnIntegerOverflow=on  InputSameDT=on  OutDataTypeStr=Inherit: Same as first input
  double integrator : Subsystem
  friction : Subsystem  mask{friction=frictionB*forceCanon, yieldDispl=yieldDisplB*lengthCanon, hysteresis=0}
      mask prompts: friction "Sliding friction"; yieldDispl "Equiv. yield displacement (in)"; hysteresis "Hysteresis constant"
  mass : Constant  Value=massB*massCanon  OutDataType=sfix(16)  OutScaling=2^0
  static force : Constant  Value=staticForceB*forceCanon  OutDataType=sfix(16)  OutScaling=2^0
  term1 : Terminator
  unit dly : UnitDelay  SampleTime=-1
  unit dly1 : UnitDelay  SampleTime=-1
  veloc units : Gain  Gain=1/velocCanon  ParameterDataType=sfix(16)  ParameterScaling=2^0  OutDataType=sfix(16)  OutScaling=2^0  SaturateOnIntegerOverflow=on  OutDataTypeStr=Inherit: Same as input  ParamDataTypeStr=Inherit: Same as input
  displ : Outport  OutDataType=sfix(16)  OutScaling=2^0
  veloc : Outport  Port=2  OutDataType=sfix(16)  OutScaling=2^0
  tag scope: ch4a=global
  wires:
  friction/1(force) -> Sum/2  "friction force"
  veloc units/1 -> veloc/1
  Sum/1 -> div/1  "inertial force"
  force/1 -> Sum/1  "total force"
  mass/1 -> div/2
  double integrator/3(acc) -> term1/1
  div/1 -> double integrator/1(accel)
  double integrator/1(displ) -> displ/1, unit dly/1
  double integrator/2(veloc) -> veloc units/1, friction/1(veloc), unit dly1/1
  static force/1 -> Sum/5  "static force"
  damper/1 -> Sum/4  "damper force"
  unit dly1/1 -> damper/1
  [ch4b] -> Sum/3  "spring force"
  unit dly/1 -> [ch4a]

== system Test_SimFEAdapter/model/ActuatorPayloadMdl/dynamic short channel #1/actuator/valve  model ==
  note: Auxiliary diagnostic output vector:
      | 1:   valve opening
      | 2:   C1 pressure
      | 3:   C2 pressure
      | 4:   delta pressure
      | 5:   force
      | 6:   velocity
      | 7:   C1 flow
      | 8:   C2 flow
      | 9:   total flow
      | 10: kinematic flow
      | 11: compressibility flow
      | 12: leakage flow
  note: Note: "1" and "2" denote actuator
      | cylinders on either side of the
      | actuator piston.  With positive
      | valve drive, oil is ported into
      | cylinder 1, resulting in positive
      | displacement.
  note: Parameter vector:
      | 1:   oil bulk modulus (force/displ^2)
      | 2:   servovalve delay (sec)
      | 3:   servovalve overlap
      | 4:   rated pressure (force/displ^2)
      | 5:   rated flow at rated pressure (displ^3/sec)
      | 6:   nominal flow at rated pressure (displ^3/sec)
      | 7:   actuator piston area 1 (displ^2)
      | 8:   actuator piston area 2 (displ^2)
      | 9:   actuator usable stroke 1 (displ)
      | 10: actuator usable stroke 2 (displ)
      | 11: actuator end cushion length 1 (displ)
      | 12: actuator end cushion length 2 (displ)
      | 13: actuator parasitic damping factor
      | 14: cross-chamber leakage factor (flow/press)
      | 15: ratio port openings according to area
      | 16: sample period (sec)
      |
      | Conversion factors used for converting
      | signals from external (user) to internal
      | (canonical) units:
      |
      | 17: displacement
      | 18: velocity
      | 19: force
      | 20: pressure
      | 21: flow
  cmd : Inport  OutDataType=sfix(16)  OutScaling=2^0
  displ : Inport  Port=2  OutDataType=sfix(16)  OutScaling=2^0
  veloc : Inport  Port=3  OutDataType=sfix(16)  OutScaling=2^0
  spl press : Inport  Port=4  OutDataType=sfix(16)  OutScaling=2^0
  rtn press : Inport  Port=5  OutDataType=sfix(16)  OutScaling=2^0
  abs : Abs  SaturateOnIntegerOverflow=on
  actuator : S-Function  FunctionName=actuator  Parameters=actParamsA  EnableBusSupport=off
  total flow sel : Selector  InputPortWidth=12  IndexOptions=Index vector (dialog)  Indices=9  OutputSizes=1
  force : Outport  OutDataType=sfix(16)  OutScaling=2^0
  flow : Outport  Port=2  OutDataType=sfix(16)  OutScaling=2^0
  wires:
  abs/1 -> flow/1
  actuator/2 -> total flow sel/1
  total flow sel/1 -> abs/1
  spl press/1 -> actuator/4
  rtn press/1 -> actuator/5
  cmd/1 -> actuator/1
  actuator/1 -> force/1
  displ/1 -> actuator/2
  veloc/1 -> actuator/3

== system Test_SimFEAdapter/model/ActuatorPayloadMdl/dynamic short channel #1/payload ==
  force : Inport  OutDataType=sfix(16)  OutScaling=2^0
  Sum : Sum  Inputs=+----  OutDataType=sfix(16)  OutScaling=2^0  SaturateOnIntegerOverflow=on  InputSameDT=on  OutDataTypeStr=Inherit: Same as first input
  damper : Gain  Gain=damperA*damperCanon  ParameterDataType=sfix(16)  ParameterScaling=2^0  OutDataType=sfix(16)  OutScaling=2^0  SaturateOnIntegerOverflow=on  OutDataTypeStr=Inherit: Same as input  ParamDataTypeStr=Inherit: Same as input
  div : Product  Inputs=*/  OutDataType=sfix(16)  OutScaling=2^0  SaturateOnIntegerOverflow=on  InputSameDT=on  OutDataTypeStr=Inherit: Same as first input
  double integrator : Subsystem
  friction : Subsystem  mask{friction=frictionA*forceCanon, yieldDispl=yieldDisplA*lengthCanon, hysteresis=0}
      mask prompts: friction "Sliding friction"; yieldDispl "Equiv. yield displacement (in)"; hysteresis "Hysteresis constant"
  mass : Constant  Value=massA*massCanon  OutDataType=sfix(16)  OutScaling=2^0
  static force : Constant  Value=staticForceA*forceCanon  OutDataType=sfix(16)  OutScaling=2^0
  term1 : Terminator
  unit dly : UnitDelay  SampleTime=-1
  unit dly1 : UnitDelay  SampleTime=-1
  veloc units : Gain  Gain=1/velocCanon  ParameterDataType=sfix(16)  ParameterScaling=2^0  OutDataType=sfix(16)  OutScaling=2^0  SaturateOnIntegerOverflow=on  OutDataTypeStr=Inherit: Same as input  ParamDataTypeStr=Inherit: Same as input
  displ : Outport  OutDataType=sfix(16)  OutScaling=2^0
  veloc : Outport  Port=2  OutDataType=sfix(16)  OutScaling=2^0
  tag scope: ch1a=global
  wires:
  friction/1(force) -> Sum/2  "friction force"
  veloc units/1 -> veloc/1
  Sum/1 -> div/1  "inertial force"
  force/1 -> Sum/1  "total force"
  mass/1 -> div/2
  double integrator/3(acc) -> term1/1
  div/1 -> double integrator/1(accel)
  double integrator/1(displ) -> displ/1, unit dly/1
  double integrator/2(veloc) -> veloc units/1, friction/1(veloc), unit dly1/1
  static force/1 -> Sum/5  "static force"
  damper/1 -> Sum/4  "damper force"
  unit dly1/1 -> damper/1
  [ch1b] -> Sum/3  "spring force"
  unit dly/1 -> [ch1a]

== system Test_SimFEAdapter/model/ActuatorPayloadMdl/dynamic short channel #2/actuator/valve  model ==
  note: Auxiliary diagnostic output vector:
      | 1:   valve opening
      | 2:   C1 pressure
      | 3:   C2 pressure
      | 4:   delta pressure
      | 5:   force
      | 6:   velocity
      | 7:   C1 flow
      | 8:   C2 flow
      | 9:   total flow
      | 10: kinematic flow
      | 11: compressibility flow
      | 12: leakage flow
  note: Note: "1" and "2" denote actuator
      | cylinders on either side of the
      | actuator piston.  With positive
      | valve drive, oil is ported into
      | cylinder 1, resulting in positive
      | displacement.
  note: Parameter vector:
      | 1:   oil bulk modulus (force/displ^2)
      | 2:   servovalve delay (sec)
      | 3:   servovalve overlap
      | 4:   rated pressure (force/displ^2)
      | 5:   rated flow at rated pressure (displ^3/sec)
      | 6:   nominal flow at rated pressure (displ^3/sec)
      | 7:   actuator piston area 1 (displ^2)
      | 8:   actuator piston area 2 (displ^2)
      | 9:   actuator usable stroke 1 (displ)
      | 10: actuator usable stroke 2 (displ)
      | 11: actuator end cushion length 1 (displ)
      | 12: actuator end cushion length 2 (displ)
      | 13: actuator parasitic damping factor
      | 14: cross-chamber leakage factor (flow/press)
      | 15: ratio port openings according to area
      | 16: sample period (sec)
      |
      | Conversion factors used for converting
      | signals from external (user) to internal
      | (canonical) units:
      |
      | 17: displacement
      | 18: velocity
      | 19: force
      | 20: pressure
      | 21: flow
  cmd : Inport  OutDataType=sfix(16)  OutScaling=2^0
  displ : Inport  Port=2  OutDataType=sfix(16)  OutScaling=2^0
  veloc : Inport  Port=3  OutDataType=sfix(16)  OutScaling=2^0
  spl press : Inport  Port=4  OutDataType=sfix(16)  OutScaling=2^0
  rtn press : Inport  Port=5  OutDataType=sfix(16)  OutScaling=2^0
  abs : Abs  SaturateOnIntegerOverflow=on
  actuator : S-Function  FunctionName=actuator  Parameters=actParamsA  EnableBusSupport=off
  total flow sel : Selector  InputPortWidth=12  IndexOptions=Index vector (dialog)  Indices=9  OutputSizes=1
  force : Outport  OutDataType=sfix(16)  OutScaling=2^0
  flow : Outport  Port=2  OutDataType=sfix(16)  OutScaling=2^0
  wires:
  abs/1 -> flow/1
  actuator/2 -> total flow sel/1
  total flow sel/1 -> abs/1
  spl press/1 -> actuator/4
  rtn press/1 -> actuator/5
  cmd/1 -> actuator/1
  actuator/1 -> force/1
  displ/1 -> actuator/2
  veloc/1 -> actuator/3

== system Test_SimFEAdapter/model/ActuatorPayloadMdl/dynamic short channel #2/payload ==
  force : Inport  OutDataType=sfix(16)  OutScaling=2^0
  Sum : Sum  Inputs=+----  OutDataType=sfix(16)  OutScaling=2^0  SaturateOnIntegerOverflow=on  InputSameDT=on  OutDataTypeStr=Inherit: Same as first input
  damper : Gain  Gain=damperA*damperCanon  ParameterDataType=sfix(16)  ParameterScaling=2^0  OutDataType=sfix(16)  OutScaling=2^0  SaturateOnIntegerOverflow=on  OutDataTypeStr=Inherit: Same as input  ParamDataTypeStr=Inherit: Same as input
  div : Product  Inputs=*/  OutDataType=sfix(16)  OutScaling=2^0  SaturateOnIntegerOverflow=on  InputSameDT=on  OutDataTypeStr=Inherit: Same as first input
  double integrator : Subsystem
  friction : Subsystem  mask{friction=frictionA*forceCanon, yieldDispl=yieldDisplA*lengthCanon, hysteresis=0}
      mask prompts: friction "Sliding friction"; yieldDispl "Equiv. yield displacement (in)"; hysteresis "Hysteresis constant"
  mass : Constant  Value=massA*massCanon  OutDataType=sfix(16)  OutScaling=2^0
  static force : Constant  Value=staticForceA*forceCanon  OutDataType=sfix(16)  OutScaling=2^0
  term1 : Terminator
  unit dly : UnitDelay  SampleTime=-1
  unit dly1 : UnitDelay  SampleTime=-1
  veloc units : Gain  Gain=1/velocCanon  ParameterDataType=sfix(16)  ParameterScaling=2^0  OutDataType=sfix(16)  OutScaling=2^0  SaturateOnIntegerOverflow=on  OutDataTypeStr=Inherit: Same as input  ParamDataTypeStr=Inherit: Same as input
  displ : Outport  OutDataType=sfix(16)  OutScaling=2^0
  veloc : Outport  Port=2  OutDataType=sfix(16)  OutScaling=2^0
  tag scope: ch2a=global
  wires:
  friction/1(force) -> Sum/2  "friction force"
  veloc units/1 -> veloc/1
  Sum/1 -> div/1  "inertial force"
  force/1 -> Sum/1  "total force"
  mass/1 -> div/2
  double integrator/3(acc) -> term1/1
  div/1 -> double integrator/1(accel)
  double integrator/1(displ) -> displ/1, unit dly/1
  double integrator/2(veloc) -> veloc units/1, friction/1(veloc), unit dly1/1
  static force/1 -> Sum/5  "static force"
  damper/1 -> Sum/4  "damper force"
  unit dly1/1 -> damper/1
  [ch2b] -> Sum/3  "spring force"
  unit dly/1 -> [ch2a]
